simulink model "Power_Window"  (R2020b)
settings: Solver=ode45  StartTime=0.0  StopTime=inf  RelTol=1e-3
PreLoadFcn:
  | clc;
  | clearvars;
values from neighbouring files (symbols this model uses):
  Bottom_Pos = 0.0    [Window_Parameter.sldd]    (also in data.mat = 0)
  Top_Pos = 20.0    [Window_Parameter.sldd]    (also in data.mat = 20)
CloseFcn:
  | clc;
  | clearvars;
settings Model: DataDictionary=Window_Parameter.sldd  EnablePacing=on  PacingRate=0.110000  Creator=vijay jagtap  LastModifiedBy=vijay jagtap

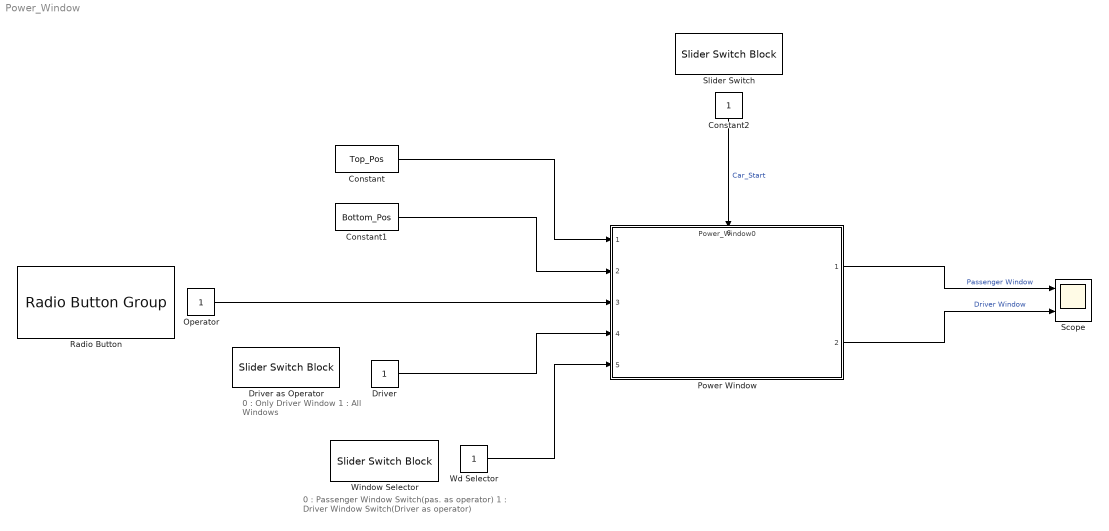
== system Power_Window ==
  note: 0 : Passenger Window Switch(pas. as operator)
      | 1 : Driver Window Switch(Driver as operator)
  note: 0 : Only Driver Window
      | 1 : All Windows
  Constant : Constant  Value=Top_Pos
  Constant1 : Constant  Value=Bottom_Pos
  Constant2 : Constant
  Driver : Constant
  Driver as Operator : SliderSwitchBlock  LabelPosition=Hide
      settings: Values={{'Off', 'On'}, [0 1]}
  Operator : Constant
  Power Window : ModelReference  ModelNameDialog=Power_Window0  ModelReferenceVersion=1.28
      settings: PortSchema="{\"entries\":[{\"content\":{\"sides\":[{\"content\":{\"connectorIds\":[\"In1\",\"In2\",\"In3\",\"In4\",\"In5\"]},\"type\":\"ConnectorPlacement.EquallySpacedRectSide\",\"uuid\":\"d9bde730-ee4f-4323-93a1-f693d508d7b7\"},{\"content\":{\"connectorIds\":[\"Out1\",\"Out2\"],\"side\":\"RIGHT\"},\"type\":\"ConnectorPlacement.EquallySpacedRectSide\",\"uuid\":\"a207c1ae-6ec1-46aa-8499-9c4b009a48e5\"},{\"content\":{\"connectorIds\":[\"In6\"],\"side\":\"TOP\"},\"type\":\"ConnectorPlacement.EquallySpacedRectSide\",\"uuid\":\"ce5b2539-f8aa-4353-8d4d-e935df1f1262\"},{\"content\":{\"connectorIds\":[],\"side\":\"HIDDEN\"},\"type\":\"ConnectorPlacement.EquallySpacedRectSide\",\"uuid\":\"5a4a55d9-9e35-4b58-8bf8-2dc8134f6554\"}]},\"type\":\"ConnectorPlacement.EquallySpacedConnector\",\"uuid\":\"ae2c6d48-90d5-47bf-9bd0-d028c3905bc5\"}],\"packageUris\":[\"http://schema.mathworks.com/mf0/Connector/R2020b\"],\"version\":\"1.0\"}"
  Radio Button : RadioButtonGroup  LabelPosition=Hide  SelectedLabel=Up  ButtonGroupName=Window Switch Operator(Driver)
      settings: Values={{'Down', 'Idle', 'Up'}, [-1 0 1]}
  Scope : Scope  NumInputPorts=2
  Slider Switch : SliderSwitchBlock  LabelPosition=Hide
      settings: Values={{'Off', 'On'}, [0 1]}
  Wd Selector : Constant
  Window Selector : SliderSwitchBlock  LabelPosition=Hide
      settings: Values={{'Off', 'On'}, [0 1]}
  wires:
  Constant/1 -> Power Window/1
  Constant1/1 -> Power Window/2
  Operator/1 -> Power Window/3
  Driver/1 -> Power Window/4
  Wd Selector/1 -> Power Window/5
  Power Window/1 -> Scope/1  "Passenger Window"
  Power Window/2 -> Scope/2  "Driver Window"
  Constant2/1 -> Power Window/6  "Car_Start"
